simulink subsystem "FromOmega2toThrust"  (R2023a)
settings: Solver=VariableStepAuto  StartTime=0.0  StopTime=10.0  RelTol=1e-3
undefined symbols (not defined in the file): HexaConstants
settings Model: Creator=Dell  LastModifiedBy=danie

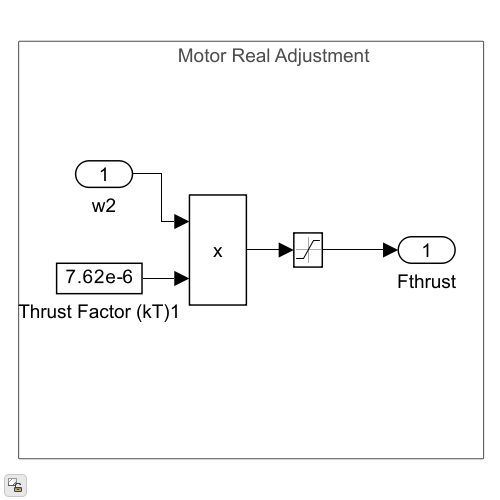
[thumbnail: Simulink's stored preview of the top-level diagram]
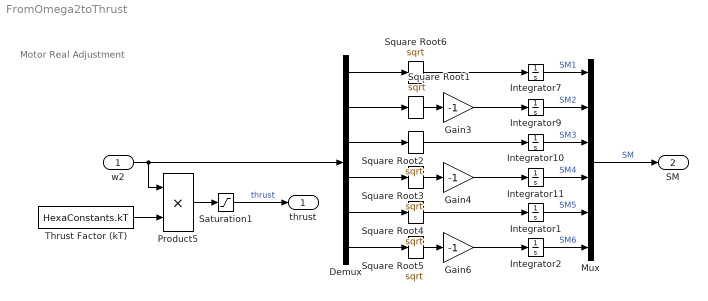
== system FromOmega2toThrust ==
  note: Motor Real Adjustment
  w2 : Inport
  Demux : Demux  Outputs=6
  Gain3 : Gain  Gain=-1
  Gain4 : Gain  Gain=-1
  Gain6 : Gain  Gain=-1
  Integrator{1..2,7,9..11} (6 alike) : Integrator
  Mux : Mux  Inputs=6
  Product5 : Product
  Saturation1 : Saturate  UpperLimit=7  LowerLimit=0
  Square Root{1..6} (6 alike) : Sqrt
  Thrust Factor (kT) : Constant  Value=HexaConstants.kT
  thrust : Outport
  SM : Outport  Port=2
  wires:
  Product5/1 -> Saturation1/1
  Thrust Factor (kT)/1 -> Product5/2
  Saturation1/1 -> thrust/1  "thrust"
  w2/1 -> Product5/1, Demux/1
  Demux/2 -> Square Root1/1
  Mux/1 -> SM/1  "SM"
  Demux/3 -> Square Root2/1
  Gain4/1 -> Integrator11/1
  Integrator2/1 -> Mux/6  "SM6"
  Integrator10/1 -> Mux/3  "SM3"
  Gain6/1 -> Integrator2/1
  Gain3/1 -> Integrator9/1
  Integrator11/1 -> Mux/4  "SM4"
  Demux/6 -> Square Root5/1
  Integrator7/1 -> Mux/1  "SM1"
  Demux/5 -> Square Root4/1
  Demux/4 -> Square Root3/1
  Integrator9/1 -> Mux/2  "SM2"
  Integrator1/1 -> Mux/5  "SM5"
  Demux/1 -> Square Root6/1
  Square Root6/1 -> Integrator7/1
  Square Root1/1 -> Gain3/1
  Square Root2/1 -> Integrator10/1
  Square Root3/1 -> Gain4/1
  Square Root4/1 -> Integrator1/1
  Square Root5/1 -> Gain6/1
